simulink model "p5p5e"  (Simulink 8.9)
settings: Solver=ode45  StartTime=0.0  StopTime=1000  RelTol=1e-3  EnableMultiTasking=on
values from neighbouring files (symbols this model uses):
  Kpd = 0.84    [P5p5d.m]    (also in P5p5e.m)
  Td = T    (= 72.52)    [P5p5d.m]    (also in P5p5e.m)
  Tf = 8.36    [P5p5d.m]    (also in P5p5e.m)
  timeSample = 1/10    (= 0.1)    [P5p5c.m]    (also in P5p5d.m; P5p5e.m)
libraries: simulink_extras x6, simulink x2
settings Model: Creator=markh  LastModifiedBy=nicholao
settings DataIOCC: SignalLoggingName=sigsOut
settings OptimizationCC: InitFltsAndDblsToZero=on
settings DebuggingCC: SaveWithParameterizedLinksMsg=none  SignalResolutionControl=TryResolveAllWithWarning  MultiTaskDSMMsg=warning  MultiTaskCondExecSysMsg=none
settings HardwareCC: TargetUnknown=on
settings GRTTargetCC: TargetFcnLib=ansi_tfl_tmw.mat

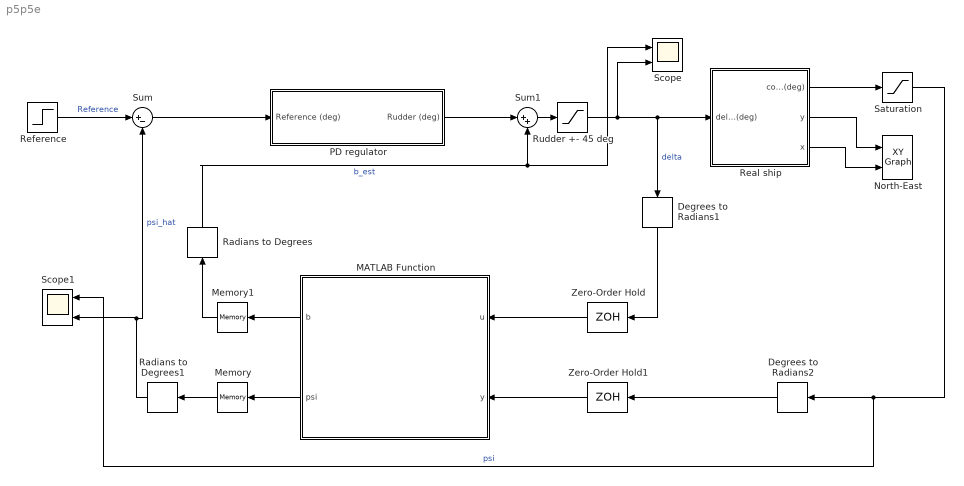
== system p5p5e ==
  Degrees to Radians1 : simulink_extras/Transformations/Degrees to Radians
  Degrees to Radians2 : simulink_extras/Transformations/Degrees to Radians
  MATLAB Function : MATLAB Function  TreatAsAtomicUnit=on
  Memory : Memory
  Memory1 : Memory
  North-East : simulink/Sinks/XY Graph  xmin=-5000  xmax=6000  ymin=-5000  ymax=5000  st=-1
  PD regulator : Subsystem
  Radians to Degrees : simulink_extras/Transformations/Radians to Degrees
  Radians to Degrees1 : simulink_extras/Transformations/Radians to Degrees
  Real ship : Subsystem  mask(Simple shipmodel for a cargo ship){noise=on, current=on, logic=on}
      mask prompts: noise "measurement noise"; logic "waves"
      mask help:
      | Measurement noise:
      | 	checked = noise on
      | 	unchecked = noise off
      |
      | Current:
      | 	checked = current on
      | 	unchecked = current off
      |
      | Waves:
      | 	checked = waves on
      | 	unchecked = waves off
      |
      | Author: Jørgen Spjøtvold, 9/10-2003
      | TTK 4115 Linear system theory.
      | Modified by Jostein Bakkeheim 26/10-2006
  Reference : Step  Time=5  After=30  SampleTime=0
  "Rudder +- 45 deg " : Saturate  UpperLimit=45  LowerLimit=-45
  Saturation : Saturate  UpperLimit=35  LowerLimit=-35
  Scope : Scope  NumInputPorts=2
  Scope1 : Scope  NumInputPorts=2
  Sum : Sum  Inputs=|+-
  Sum1 : Sum  Inputs=|++
  Zero-Order Hold : ZeroOrderHold  SampleTime=timeSample
  Zero-Order Hold1 : ZeroOrderHold  SampleTime=timeSample
  wires:
  Real ship/3(x) -> North-East/2
  Real ship/2(y) -> North-East/1
  Real ship/1(compass (deg)) -> Saturation/1
  Zero-Order Hold/1 -> MATLAB Function/1(u)
  Zero-Order Hold1/1 -> MATLAB Function/2(y)
  MATLAB Function/1(b) -> Memory1/1
  MATLAB Function/2(psi) -> Memory/1
  Sum1/1 -> "Rudder +- 45 deg "/1
  Saturation/1 -> Scope1/1, Degrees to Radians2/1  "psi"
  Memory1/1 -> Radians to Degrees/1
  Sum/1 -> PD regulator/1(Reference (deg))
  PD regulator/1(Rudder (deg)) -> Sum1/1
  Memory/1 -> Radians to Degrees1/1
  "Rudder +- 45 deg "/1 -> Scope/2, Degrees to Radians1/1, Real ship/1(delta (deg))  "delta"
  Degrees to Radians2/1 -> Zero-Order Hold1/1
  Degrees to Radians1/1 -> Zero-Order Hold/1
  Radians to Degrees/1 -> Scope/1, Sum1/2  "b_est"
  Radians to Degrees1/1 -> Sum/2, Scope1/2  "psi_hat"
  Reference/1 -> Sum/1  "Reference"

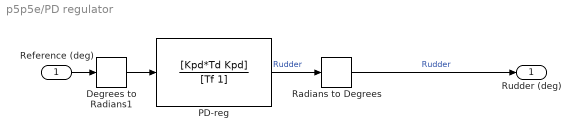
== system p5p5e/PD regulator ==
  Reference (deg) : Inport
  Degrees to Radians1 : simulink_extras/Transformations/Degrees to Radians
  PD-reg : TransferFcn  Numerator=[Kpd*Td Kpd]  Denominator=[Tf 1]
  Radians to Degrees : simulink_extras/Transformations/Radians to Degrees
  Rudder (deg) : Outport
  wires:
  Degrees to Radians1/1 -> PD-reg/1
  Radians to Degrees/1 -> Rudder (deg)/1  "Rudder"
  Reference (deg)/1 -> Degrees to Radians1/1
  PD-reg/1 -> Radians to Degrees/1  "Rudder"

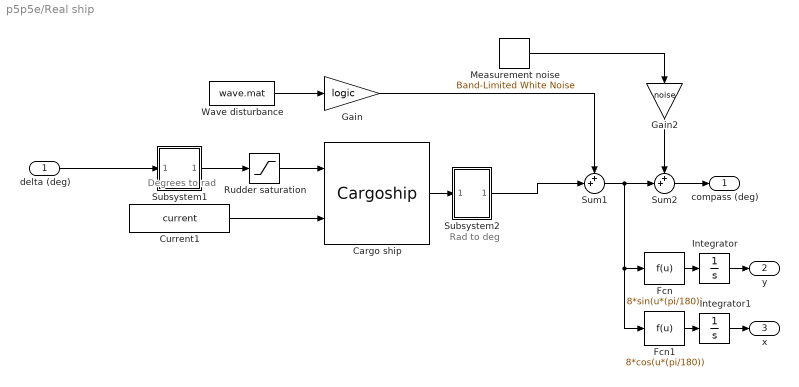
== system p5p5e/Real ship ==
  note: Degrees to rad
  note: Rad to deg
  delta (deg) : Inport
  Cargo ship : S-Function  FunctionName=Cargoship  SFunctionDeploymentMode=off  EnableBusSupport=off  mask(Cargo ship){}
      mask help:
      | S-function which simulates a cargo ship.
      |
      | Author: Jørgen Spjøtvold
      | 20.10-2003
      | Modified by Jostein Bakkeheim 27.10.2006
  Current1 : Constant  Value=current
  Fcn : Fcn  Expr=8*sin(u*(pi/180))
  Fcn1 : Fcn  Expr=8*cos(u*(pi/180))
  Gain : Gain  Gain=logic  SaturateOnIntegerOverflow=on  OutDataTypeStr=Inherit: Same as input  ParamDataTypeStr=Inherit: Same as input
  Gain2 : Gain  Gain=noise  SaturateOnIntegerOverflow=on  OutDataTypeStr=Inherit: Same as input  ParamDataTypeStr=Inherit: Same as input
  Integrator : Integrator
  Integrator1 : Integrator
  Measurement noise : simulink/Sources/Band-Limited White Noise  Cov=[0.001]  Ts=.5  seed=[23341]
  Rudder saturation : Saturate  UpperLimit=45*(pi/180)  LowerLimit=-45*(pi/180)
  Subsystem1 : Subsystem  mask(degrees to radians){}
      mask help: Converts degrees to radians
      mask Display: fprintf('D2R');
  Subsystem2 : Subsystem  mask(radians to degrees){}
      mask help: Converts radians to degrees
      mask Display: fprintf('R2D');
  Sum1 : Sum  Inputs=++|  SaturateOnIntegerOverflow=on
  Sum2 : Sum  Inputs=++|  SaturateOnIntegerOverflow=on
  Wave disturbance : FromFile  FileName=wave.mat  SampleTime=0
  compass (deg) : Outport
  y : Outport  Port=2
  x : Outport  Port=3
  wires:
  delta (deg)/1 -> Subsystem1/1(In1)
  Fcn/1 -> Integrator/1
  Integrator/1 -> y/1
  Fcn1/1 -> Integrator1/1
  Integrator1/1 -> x/1
  Wave disturbance/1 -> Gain/1
  Subsystem2/1(Out1) -> Sum1/2
  Sum1/1 -> Fcn/1, Fcn1/1, Sum2/2
  Cargo ship/1 -> Subsystem2/1(In1)
  Subsystem1/1(Out1) -> Rudder saturation/1
  Rudder saturation/1 -> Cargo ship/1
  Sum2/1 -> compass (deg)/1
  Measurement noise/1 -> Gain2/1
  Gain2/1 -> Sum2/1
  Current1/1 -> Cargo ship/2
  Gain/1 -> Sum1/1

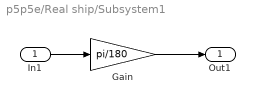
== system p5p5e/Real ship/Subsystem1 ==
  In1 : Inport
  Gain : Gain  Gain=pi/180  SaturateOnIntegerOverflow=on  OutDataTypeStr=Inherit: Same as input  ParamDataTypeStr=Inherit: Same as input
  Out1 : Outport
  wires:
  Gain/1 -> Out1/1
  In1/1 -> Gain/1

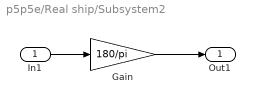
== system p5p5e/Real ship/Subsystem2 ==
  In1 : Inport
  Gain : Gain  Gain=180/pi  SaturateOnIntegerOverflow=on  OutDataTypeStr=Inherit: Same as input  ParamDataTypeStr=Inherit: Same as input
  Out1 : Outport
  wires:
  Gain/1 -> Out1/1
  In1/1 -> Gain/1

== matlab function MATLAB Function ==
  data: u input double; b output double; y input double; psi output double; dataStruct parameter double
function [b, psi] = Kalman(u, y, dataStruct)

persistent init_flag A B C E Q R P_ x_


if isempty(init_flag)
    % Initialization for system
    init_flag = 1;
    
    [A,B,C,E,Q,R,P_,x_] = deal(dataStruct.A, dataStruct.B, dataStruct.C, ...
                            dataStruct.E, dataStruct.Q, dataStruct.R,...
                            dataStruct.P_, dataStruct.x_);
end

I = eye(5);

K =  (P_*C')*inv((C*P_*C'+R));

x = x_ + K*(y-C*x_);

P = (I-K*C)*P_*(I-K*C)'+K*R*K';

x_ = A*x + B*u;

P_ = A*P*A'+E*Q*E';

b = x(5);
psi = x(3);
end
